simulink model "simulare_lab4"  (R2024b)
settings: Solver=VariableStepAuto  StartTime=0.0  StopTime=0.3  RelTol=1e-3
values from neighbouring files (symbols this model uses):
  A = [-Ra/La, -K/La; K/J, 0;]    [Lab4.m]    (also in Lab4_recapitulare.m)
  B = [1/La, 0; 0, -1/J]    [Lab4.m]    (also in Lab4_recapitulare.m)
  C = [1, 0; 0, 1]    [Lab4.m]    (also in Lab4_recapitulare.m)
  D = [0, 0; 0, 0]    [Lab4.m]    (also in Lab4_recapitulare.m)
undefined symbols (not defined in the file or in its folder): dens1, dens2, nums1, nums2
settings Model: Creator=akopo  LastModifiedBy=akopo

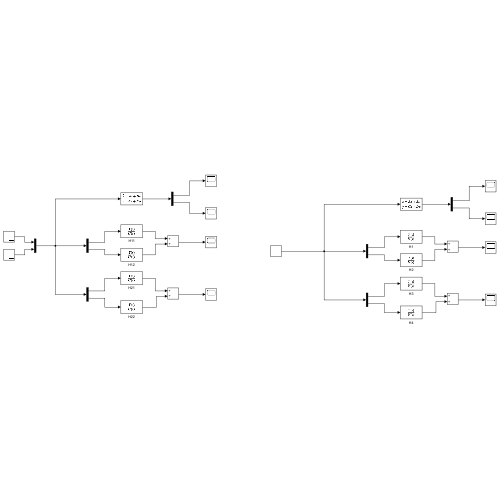
[thumbnail: Simulink's stored preview of the top-level diagram]
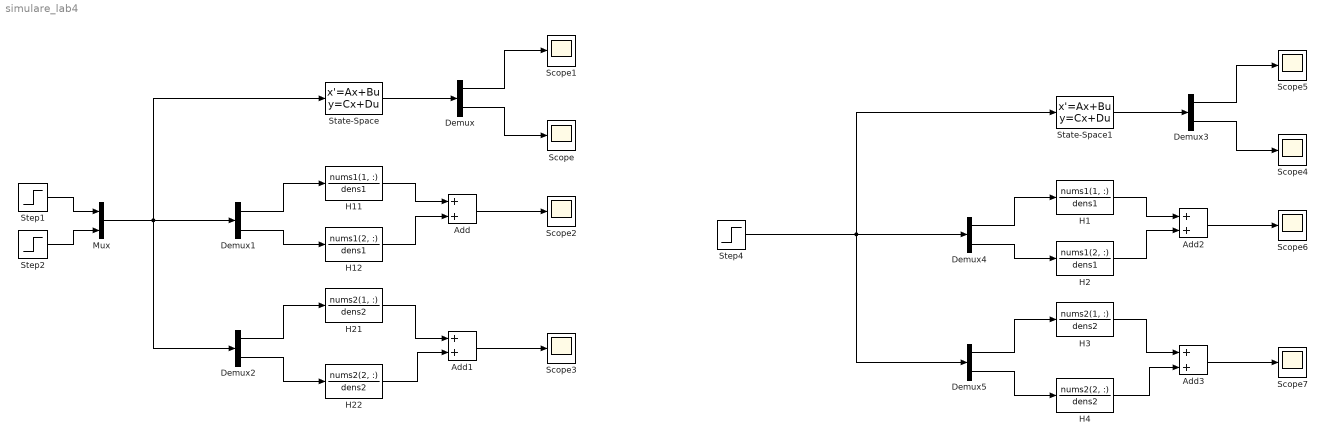
== system simulare_lab4 ==
  Add{,1..3} (4 alike) : Sum
  Demux{,1..5} (6 alike) : Demux  Outputs=2
  H1 : TransferFcn  Numerator=nums1(1, :)  Denominator=dens1
  H11 : TransferFcn  Numerator=nums1(1, :)  Denominator=dens1
  H12 : TransferFcn  Numerator=nums1(2, :)  Denominator=dens1
  H2 : TransferFcn  Numerator=nums1(2, :)  Denominator=dens1
  H21 : TransferFcn  Numerator=nums2(1, :)  Denominator=dens2
  H22 : TransferFcn  Numerator=nums2(2, :)  Denominator=dens2
  H3 : TransferFcn  Numerator=nums2(1, :)  Denominator=dens2
  H4 : TransferFcn  Numerator=nums2(2, :)  Denominator=dens2
  Mux : Mux  Inputs=2
  Scope{,1..7} (8 alike) : Scope
  State-Space : StateSpace  A=A  B=B  C=C  D=D  InitialCondition=0
  State-Space1 : StateSpace  A=A  B=B  C=C  D=D  InitialCondition=0
  Step1 : Step  Time=0.1  Before=24  After=0  SampleTime=0
  Step2 : Step  Time=0.2  Before=0.04  After=-0.24  SampleTime=0
  Step4 : Step  Time=0  After=[24; 0.04]  SampleTime=0
  wires:
  State-Space/1 -> Demux/1
  Demux/2 -> Scope/1
  Demux/1 -> Scope1/1
  Demux1/1 -> H11/1
  Demux1/2 -> H12/1
  Demux2/1 -> H21/1
  Demux2/2 -> H22/1
  Add/1 -> Scope2/1
  Add1/1 -> Scope3/1
  H12/1 -> Add/2
  H11/1 -> Add/1
  H21/1 -> Add1/1
  H22/1 -> Add1/2
  Mux/1 -> Demux2/1, State-Space/1, Demux1/1
  Step1/1 -> Mux/1
  Step2/1 -> Mux/2
  H2/1 -> Add2/2
  Demux5/1 -> H3/1
  Demux5/2 -> H4/1
  H1/1 -> Add2/1
  Add2/1 -> Scope6/1
  Demux3/1 -> Scope5/1
  Demux4/1 -> H1/1
  Demux3/2 -> Scope4/1
  H3/1 -> Add3/1
  Step4/1 -> Demux4/1, Demux5/1, State-Space1/1
  State-Space1/1 -> Demux3/1
  Demux4/2 -> H2/1
  Add3/1 -> Scope7/1
  H4/1 -> Add3/2
